simulink library "fcw"  (Simulink 8.1)
settings: Solver=ode45  StartTime=0.0  StopTime=10.0  RelTol=1e-3
undefined symbols (not defined in the file or in its folder): KFCW_BrakePreFillTimer_ms, KFCW_HapticOnTimer_ms
libraries: afa x1, scw x1
settings Model: Creator=xsellart  LastModifiedBy=tescamilla

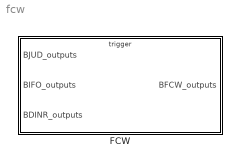
== system fcw ==
  FCW : Subsystem  TreatAsAtomicUnit=on

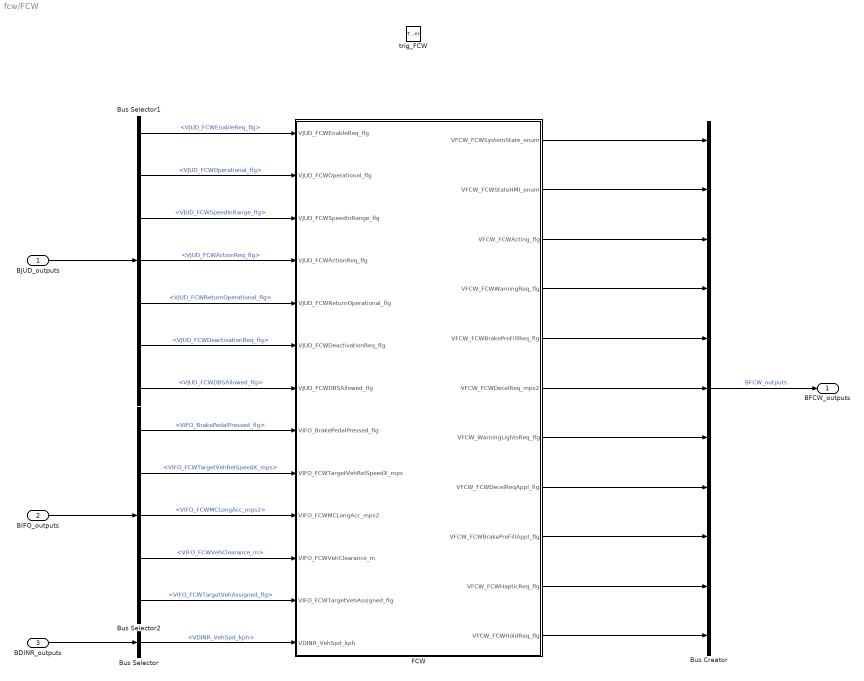
== system fcw/FCW ==
  BJUD_outputs : Inport  OutDataTypeStr=Bus: BJUD_outputs
  BIFO_outputs : Inport  Port=2  OutDataTypeStr=Bus: BIFO_outputs
  BDINR_outputs : Inport  Port=3  OutDataTypeStr=Bus: BDINR_outputs
  trig_FCW : TriggerPort  TriggerType=function-call
      settings: AttributesFormatString=State = %<StatesWhenEnabling>
  Bus Creator : BusCreator  Inputs=11  OutDataTypeStr=Bus: BFCW_outputs
  Bus Selector : BusSelector  OutputSignals=VDINR_VehSpd_kph
  Bus Selector1 : BusSelector  OutputSignals=VJUD_FCWEnableReq_flg,VJUD_FCWOperational_flg,VJUD_FCWSpeedInRange_flg,VJUD_FCWActionReq_flg,VJUD_FCWReturnOperational_flg,VJUD_FCWDeactivationReq_flg,VJUD_FCWDBSAllowed_flg
  Bus Selector2 : BusSelector  OutputSignals=VIFO_BrakePedalPressed_flg,VIFO_FCWTargetVehRelSpeedX_mps,VIFO_FCWMCLongAcc_mps2,VIFO_FCWVehClearance_m,VIFO_FCWTargetVehAssigned_flg
  FCW : Subsystem
  BFCW_outputs : Outport  OutDataTypeStr=Bus: BFCW_outputs
  wires:
  BDINR_outputs/1 -> Bus Selector/1
  Bus Creator/1 -> BFCW_outputs/1  "BFCW_outputs"
  FCW/1(VFCW_FCWSystemState_enum) -> Bus Creator/1
  FCW/2(VFCW_FCWStateHMI_enum) -> Bus Creator/2
  FCW/3(VFCW_FCWActing_flg) -> Bus Creator/3
  FCW/7(VFCW_WarningLightsReq_flg) -> Bus Creator/7
  FCW/6(VFCW_FCWDecelReq_mps2) -> Bus Creator/6
  FCW/5(VFCW_FCWBrakePreFillReq_flg) -> Bus Creator/5
  FCW/4(VFCW_FCWWarningReq_flg) -> Bus Creator/4
  Bus Selector/1 -> FCW/13(VDINR_VehSpd_kph)  "<VDINR_VehSpd_kph>"
  Bus Selector1/1 -> FCW/1(VJUD_FCWEnableReq_flg)  "<VJUD_FCWEnableReq_flg>"
  Bus Selector1/2 -> FCW/2(VJUD_FCWOperational_flg)  "<VJUD_FCWOperational_flg>"
  Bus Selector1/3 -> FCW/3(VJUD_FCWSpeedInRange_flg)  "<VJUD_FCWSpeedInRange_flg>"
  Bus Selector1/4 -> FCW/4(VJUD_FCWActionReq_flg)  "<VJUD_FCWActionReq_flg>"
  Bus Selector1/6 -> FCW/6(VJUD_FCWDeactivationReq_flg)  "<VJUD_FCWDeactivationReq_flg>"
  Bus Selector1/7 -> FCW/7(VJUD_FCWDBSAllowed_flg)  "<VJUD_FCWDBSAllowed_flg>"
  Bus Selector2/1 -> FCW/8(VIFO_BrakePedalPressed_flg)  "<VIFO_BrakePedalPressed_flg>"
  BJUD_outputs/1 -> Bus Selector1/1
  Bus Selector2/2 -> FCW/9(VIFO_FCWTargetVehRelSpeedX_mps)  "<VIFO_FCWTargetVehRelSpeedX_mps>"
  BIFO_outputs/1 -> Bus Selector2/1
  FCW/11(VFCW_FCWHoldReq_flg) -> Bus Creator/11
  FCW/10(VFCW_FCWHapticReq_flg) -> Bus Creator/10
  FCW/9(VFCW_FCWBrakePreFillAppl_flg) -> Bus Creator/9
  FCW/8(VFCW_FCWDecelReqAppl_flg) -> Bus Creator/8
  Bus Selector1/5 -> FCW/5(VJUD_FCWReturnOperational_flg)  "<VJUD_FCWReturnOperational_flg>"
  Bus Selector2/3 -> FCW/10(VIFO_FCWMCLongAcc_mps2)  "<VIFO_FCWMCLongAcc_mps2>"
  Bus Selector2/4 -> FCW/11(VIFO_FCWVehClearance_m)  "<VIFO_FCWVehClearance_m>"
  Bus Selector2/5 -> FCW/12(VIFO_FCWTargetVehAssigned_flg)  "<VIFO_FCWTargetVehAssigned_flg>"

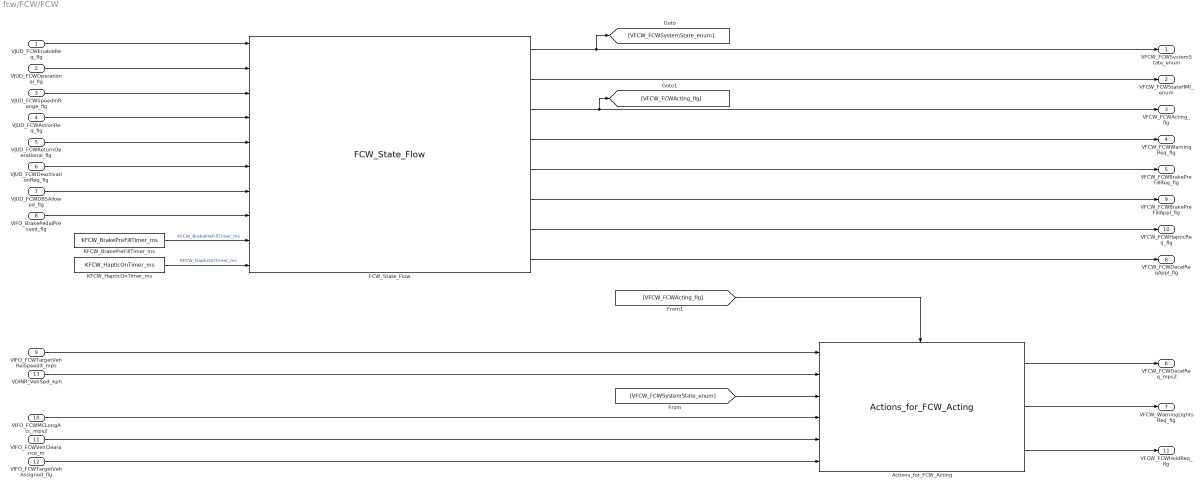
== system fcw/FCW/FCW ==
  VJUD_FCWEnableReq_flg : Inport
  VJUD_FCWOperational_flg : Inport  Port=2
  VJUD_FCWSpeedInRange_flg : Inport  Port=3
  VJUD_FCWActionReq_flg : Inport  Port=4
  VJUD_FCWReturnOperational_flg : Inport  Port=5
  VJUD_FCWDeactivationReq_flg : Inport  Port=6
  VJUD_FCWDBSAllowed_flg : Inport  Port=7
  VIFO_BrakePedalPressed_flg : Inport  Port=8
  VIFO_FCWTargetVehRelSpeedX_mps : Inport  Port=9
  VIFO_FCWMCLongAcc_mps2 : Inport  Port=10
  VIFO_FCWVehClearance_m : Inport  Port=11
  VIFO_FCWTargetVehAssigned_flg : Inport  Port=12
  VDINR_VehSpd_kph : Inport  Port=13
  Actions_for_FCW_Acting : afa/Actions_for_FCW_Acting
  FCW_State_Flow : scw/FCW_State_Flow
  KFCW_BrakePreFillTimer_ms : Constant  Value=KFCW_BrakePreFillTimer_ms
  KFCW_HapticOnTimer_ms : Constant  Value=KFCW_HapticOnTimer_ms
  VFCW_FCWSystemState_enum : Outport
  VFCW_FCWStateHMI_enum : Outport  Port=2
  VFCW_FCWActing_flg : Outport  Port=3
  VFCW_FCWWarningReq_flg : Outport  Port=4
  VFCW_FCWBrakePreFillReq_flg : Outport  Port=5
  VFCW_FCWDecelReq_mps2 : Outport  Port=6
  VFCW_WarningLightsReq_flg : Outport  Port=7
  VFCW_FCWDecelReqAppl_flg : Outport  Port=8
  VFCW_FCWBrakePreFillAppl_flg : Outport  Port=9
  VFCW_FCWHapticReq_flg : Outport  Port=10
  VFCW_FCWHoldReq_flg : Outport  Port=11
  wires:
  KFCW_HapticOnTimer_ms/1 -> FCW_State_Flow/10  "KFCW_HapticOnTimer_ms"
  KFCW_BrakePreFillTimer_ms/1 -> FCW_State_Flow/9  "KFCW_BrakePreFillTimer_ms"
  VJUD_FCWSpeedInRange_flg/1 -> FCW_State_Flow/3
  VDINR_VehSpd_kph/1 -> Actions_for_FCW_Acting/2
  Actions_for_FCW_Acting/1 -> VFCW_FCWDecelReq_mps2/1
  Actions_for_FCW_Acting/2 -> VFCW_WarningLightsReq_flg/1
  FCW_State_Flow/1 -> [VFCW_FCWSystemState_enum], VFCW_FCWSystemState_enum/1
  FCW_State_Flow/2 -> VFCW_FCWStateHMI_enum/1
  FCW_State_Flow/3 -> [VFCW_FCWActing_flg], VFCW_FCWActing_flg/1
  FCW_State_Flow/4 -> VFCW_FCWWarningReq_flg/1
  FCW_State_Flow/5 -> VFCW_FCWBrakePreFillReq_flg/1
  VJUD_FCWEnableReq_flg/1 -> FCW_State_Flow/1
  VJUD_FCWOperational_flg/1 -> FCW_State_Flow/2
  VJUD_FCWActionReq_flg/1 -> FCW_State_Flow/4
  VJUD_FCWDeactivationReq_flg/1 -> FCW_State_Flow/6
  VJUD_FCWDBSAllowed_flg/1 -> FCW_State_Flow/7
  VIFO_BrakePedalPressed_flg/1 -> FCW_State_Flow/8
  VIFO_FCWTargetVehRelSpeedX_mps/1 -> Actions_for_FCW_Acting/1
  FCW_State_Flow/6 -> VFCW_FCWBrakePreFillAppl_flg/1
  FCW_State_Flow/7 -> VFCW_FCWHapticReq_flg/1
  FCW_State_Flow/8 -> VFCW_FCWDecelReqAppl_flg/1
  Actions_for_FCW_Acting/3 -> VFCW_FCWHoldReq_flg/1
  [VFCW_FCWSystemState_enum] -> Actions_for_FCW_Acting/3
  [VFCW_FCWActing_flg] -> Actions_for_FCW_Acting/Enable
  VJUD_FCWReturnOperational_flg/1 -> FCW_State_Flow/5
  VIFO_FCWMCLongAcc_mps2/1 -> Actions_for_FCW_Acting/4
  VIFO_FCWVehClearance_m/1 -> Actions_for_FCW_Acting/5
  VIFO_FCWTargetVehAssigned_flg/1 -> Actions_for_FCW_Acting/6
